simulink model "AJAC_Simulation"  (R2024b)
settings: Solver=FixedStepAuto  StartTime=0.0  StopTime=1  FixedStep=0.000025  RelTol=1e-7  EnableMultiTasking=on
InitFcn:
  | Ld=5.25e-3;
  | Lq=12e-3;
  | R=0.958;
  | f=0.1827;
model workspace (MAT data in the model file):
  f = Simulink.Signal
  f.Dimensions = 1
  f.DimensionsMode = 'auto'
  f.Complexity = 'real'
  f.SampleTime = -1
  f.SamplingMode = 'auto'
  f.InitialValue = '0.1827'
  f.DataType = 'single'
libraries: slpidlib x2, mcbplantlib x1, simulink x1, spsPermanentMagnetSynchronousMachineLib x1, autolibpmsmexterior x1, spspowerguiLib x1
(part 1 of 2)
settings Model: Creator=张豪  LastModifiedBy=ergo
settings SolverCC: AutoInsertRateTranBlk=on
settings DebuggingCC: MultiTaskDSMMsg=none  UnconnectedInputMsg=warning  UnconnectedOutputMsg=warning  UnconnectedLineMsg=warning
settings ModelReferenceCC: EnableRefExpFcnMdlSchedulingChecks=on
settings RTWCC: GPUComputeCapability=3.5  DLArmComputeVersion=19.05

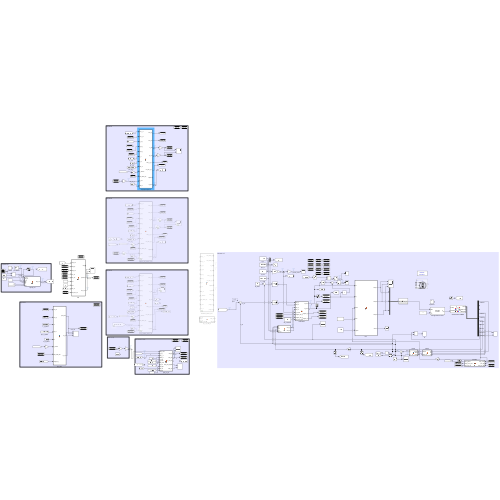
[thumbnail: Simulink's stored preview of the top-level diagram]
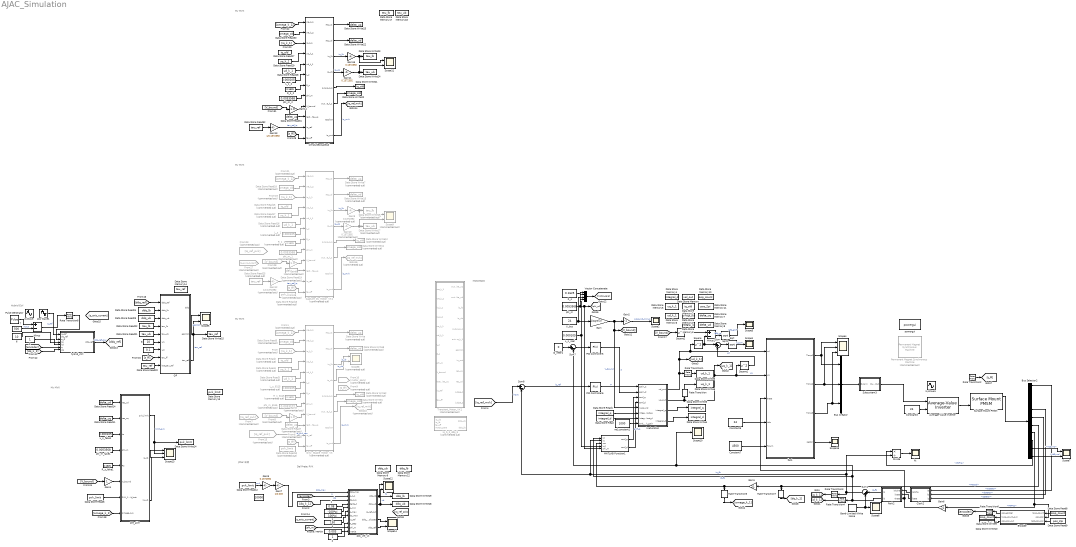
== system AJAC_Simulation ==
  note: jitter 来源
  note: Hybrid Ctrl
  note: My MVK
  note: Del Prete: PVK
  note: Motor8115
  note: My MVK
  note: My MVK
  note: My MVK
  " " : Constant  Value=10000
  "  " : Constant  Value=-100*pi
  " 1" : Constant  Value=0.08
  " 2" : Constant
  " 3" : Constant  Value=100*pi
  " 4" : Constant  Value=150
  " 5" : Constant
  " 6" : Constant  Value=10
  " 7" : Constant  Value=500
  " 8" : Constant  Value=10
  " 9" : Constant  Value=0.1
  Average-Value Inverter : mcbplantlib/Average-Value Inverter
  Band-Limited White Noise : simulink/Sources/Band-Limited White Noise  Cov=[0.0000002]  Ts=0.000025  seed=[23341]
  Bus Creator : BusCreator  Inputs=3
  Bus Selector2 : BusSelector  OutputSignals=IaStator,IqSync,IdSync,IbStator,IcStator,MtrSpd,MtrPos,MtrTrq,VqSync,VdSync
  Capture_Dy_Motor_VK1 : MATLAB Function  Commented=on  TreatAsAtomicUnit=on
  Clark2 : MATLAB Function  TreatAsAtomicUnit=on
  Constant3 : Constant  Value=24
  Constant6 : Constant  Value=24
  Constant7 : Constant  Value=4500  OutDataTypeStr=single
  Data Store Memory : DataStoreMemory  DataStoreName=vel_out  ReadBeforeWriteMsg=warning  WriteAfterWriteMsg=warning  WriteAfterReadMsg=warning  ShowAdditionalParam=off  OutDataTypeStr=double
  Data Store Memory1 : DataStoreMemory  DataStoreName=omega_old  ReadBeforeWriteMsg=warning  WriteAfterWriteMsg=warning  WriteAfterReadMsg=warning  ShowAdditionalParam=off  OutDataTypeStr=double
  Data Store Memory10 : DataStoreMemory  DataStoreName=loop_count  ReadBeforeWriteMsg=warning  WriteAfterWriteMsg=warning  WriteAfterReadMsg=warning  ShowAdditionalParam=off  OutDataTypeStr=double
  Data Store Memory11 : DataStoreMemory  DataStoreName=pos_2pi  ReadBeforeWriteMsg=warning  WriteAfterWriteMsg=warning  WriteAfterReadMsg=warning  ShowAdditionalParam=off  OutDataTypeStr=double
  Data Store Memory12 : DataStoreMemory  DataStoreName=ddq_lb  ReadBeforeWriteMsg=warning  WriteAfterWriteMsg=warning  WriteAfterReadMsg=warning  InitialValue=-1330  ShowAdditionalParam=off  OutDataTypeStr=double
  Data Store Memory13 : DataStoreMemory  DataStoreName=pvk_limit  ReadBeforeWriteMsg=warning  WriteAfterWriteMsg=warning  WriteAfterReadMsg=warning  ShowAdditionalParam=off  OutDataTypeStr=double
  Data Store Memory14 : DataStoreMemory  DataStoreName=tau_ref  ReadBeforeWriteMsg=warning  WriteAfterWriteMsg=warning  WriteAfterReadMsg=warning  ShowAdditionalParam=off  OutDataTypeStr=double
  Data Store Memory17 : DataStoreMemory  DataStoreName=tau_lb  ReadBeforeWriteMsg=warning  WriteAfterWriteMsg=warning  WriteAfterReadMsg=warning  InitialValue=-4  ShowAdditionalParam=off  OutDataTypeStr=double
  Data Store Memory18 : DataStoreMemory  DataStoreName=tau_ub  ReadBeforeWriteMsg=warning  WriteAfterWriteMsg=warning  WriteAfterReadMsg=warning  InitialValue=4  ShowAdditionalParam=off  OutDataTypeStr=double
  Data Store Memory2 : DataStoreMemory  DataStoreName=iq_old  ReadBeforeWriteMsg=warning  WriteAfterWriteMsg=warning  WriteAfterReadMsg=warning  ShowAdditionalParam=off  OutDataTypeStr=double
  Data Store Memory3 : DataStoreMemory  DataStoreName=integral_q  ReadBeforeWriteMsg=warning  WriteAfterWriteMsg=warning  WriteAfterReadMsg=warning  ShowAdditionalParam=off  OutDataTypeStr=double
  Data Store Memory4 : DataStoreMemory  DataStoreName=integral_d  ReadBeforeWriteMsg=warning  WriteAfterWriteMsg=warning  WriteAfterReadMsg=warning  ShowAdditionalParam=off  OutDataTypeStr=double
  Data Store Memory5 : DataStoreMemory  DataStoreName=uq_k_1  ReadBeforeWriteMsg=warning  WriteAfterWriteMsg=warning  WriteAfterReadMsg=warning  ShowAdditionalParam=off  OutDataTypeStr=double
  Data Store Memory6 : DataStoreMemory  DataStoreName=ud_k_1  ReadBeforeWriteMsg=warning  WriteAfterWriteMsg=warning  WriteAfterReadMsg=warning  ShowAdditionalParam=off  OutDataTypeStr=double
  Data Store Memory7 : DataStoreMemory  DataStoreName=delta_uq  ReadBeforeWriteMsg=warning  WriteAfterWriteMsg=warning  WriteAfterReadMsg=warning  ShowAdditionalParam=off  OutDataTypeStr=double
  Data Store Memory8 : DataStoreMemory  DataStoreName=delta_ud  ReadBeforeWriteMsg=warning  WriteAfterWriteMsg=warning  WriteAfterReadMsg=warning  ShowAdditionalParam=off  OutDataTypeStr=double
  Data Store Memory9 : DataStoreMemory  DataStoreName=ddq_ub  ReadBeforeWriteMsg=warning  WriteAfterWriteMsg=warning  WriteAfterReadMsg=warning  InitialValue=1330  ShowAdditionalParam=off  OutDataTypeStr=double
  Data Store Read : DataStoreRead  DataStoreName=integral_d  DataStoreElements=integral_d  IndexOptions=Index vector (dialog)  Indices=1  OutputSizes=1
  Data Store Read1 : DataStoreRead  DataStoreName=integral_q  DataStoreElements=integral_q  IndexOptions=Index vector (dialog)  Indices=1  OutputSizes=1
  Data Store Read10 : DataStoreRead  Commented=on  DataStoreName=pvk_limit  IndexOptions=Index vector (dialog)  Indices=1  OutputSizes=1
  Data Store Read11 : DataStoreRead  DataStoreName=delta_uq  IndexOptions=Index vector (dialog)  Indices=1  OutputSizes=1
  Data Store Read12 : DataStoreRead  DataStoreName=pvk_limit  IndexOptions=Index vector (dialog)  Indices=1  OutputSizes=1
  Data Store Read13 : DataStoreRead  Commented=on  DataStoreName=pvk_limit  IndexOptions=Index vector (dialog)  Indices=1  OutputSizes=1
  Data Store Read14 : DataStoreRead  DataStoreName=delta_ud  IndexOptions=Index vector (dialog)  Indices=1  OutputSizes=1
  Data Store Read15 : DataStoreRead  Commented=on  DataStoreName=iq_old  DataStoreElements=iq_old  IndexOptions=Index vector (dialog)  Indices=1  OutputSizes=1
  Data Store Read16 : DataStoreRead  Commented=on  DataStoreName=ud_k_1  IndexOptions=Index vector (dialog)  Indices=1  OutputSizes=1
  Data Store Read17 : DataStoreRead  Commented=on  DataStoreName=uq_k_1  IndexOptions=Index vector (dialog)  Indices=1  OutputSizes=1
  Data Store Read18 : DataStoreRead  Commented=on  DataStoreName=omega_old  IndexOptions=Index vector (dialog)  Indices=1  OutputSizes=1
  Data Store Read19 : DataStoreRead  Commented=on  DataStoreName=delta_uq  IndexOptions=Index vector (dialog)  Indices=1  OutputSizes=1
  Data Store Read2 : DataStoreRead  Commented=on  DataStoreName=iq_old  DataStoreElements=iq_old  IndexOptions=Index vector (dialog)  Indices=1  OutputSizes=1
  Data Store Read20 : DataStoreRead  DataStoreName=tau_ref  IndexOptions=Index vector (dialog)  Indices=1  OutputSizes=1
  Data Store Read21 : DataStoreRead  DataStoreName=tau_ub  IndexOptions=Index vector (dialog)  Indices=1  OutputSizes=1
  Data Store Read22 : DataStoreRead  DataStoreName=tau_lb  IndexOptions=Index vector (dialog)  Indices=1  OutputSizes=1
  Data Store Read23 : DataStoreRead  DataStoreName=ddq_ub  IndexOptions=Index vector (dialog)  Indices=1  OutputSizes=1
  Data Store Read24 : DataStoreRead  DataStoreName=ddq_lb  IndexOptions=Index vector (dialog)  Indices=1  OutputSizes=1
  Data Store Read25 : DataStoreRead  Commented=on  DataStoreName=tau_ref  IndexOptions=Index vector (dialog)  Indices=1  OutputSizes=1
  Data Store Read27 : DataStoreRead  DataStoreName=iq_old  DataStoreElements=iq_old  IndexOptions=Index vector (dialog)  Indices=1  OutputSizes=1
  Data Store Read28 : DataStoreRead  DataStoreName=ud_k_1  IndexOptions=Index vector (dialog)  Indices=1  OutputSizes=1
  Data Store Read29 : DataStoreRead  DataStoreName=uq_k_1  IndexOptions=Index vector (dialog)  Indices=1  OutputSizes=1
  Data Store Read3 : DataStoreRead  Commented=on  DataStoreName=ud_k_1  IndexOptions=Index vector (dialog)  Indices=1  OutputSizes=1
  Data Store Read30 : DataStoreRead  DataStoreName=omega_old  IndexOptions=Index vector (dialog)  Indices=1  OutputSizes=1
  Data Store Read31 : DataStoreRead  DataStoreName=delta_uq  IndexOptions=Index vector (dialog)  Indices=1  OutputSizes=1
  Data Store Read32 : DataStoreRead  DataStoreName=tau_ref  IndexOptions=Index vector (dialog)  Indices=1  OutputSizes=1
  Data Store Read4 : DataStoreRead  Commented=on  DataStoreName=uq_k_1  IndexOptions=Index vector (dialog)  Indices=1  OutputSizes=1
  Data Store Read5 : DataStoreRead  Commented=on  DataStoreName=omega_old  IndexOptions=Index vector (dialog)  Indices=1  OutputSizes=1
  Data Store Read6 : DataStoreRead  DataStoreName=pvk_limit  IndexOptions=Index vector (dialog)  Indices=1  OutputSizes=1
  Data Store Read7 : DataStoreRead  Commented=on  DataStoreName=delta_uq  IndexOptions=Index vector (dialog)  Indices=1  OutputSizes=1
  Data Store Read8 : DataStoreRead  DataStoreName=loop_count  IndexOptions=Index vector (dialog)  Indices=1  OutputSizes=1
  Data Store Read9 : DataStoreRead  DataStoreName=pos_2pi  IndexOptions=Index vector (dialog)  Indices=1  OutputSizes=1
  Data Store Write : DataStoreWrite  Commented=on  DataStoreName=delta_uq  IndexOptions=Index vector (dialog)  Indices=1  OutputSizes=1
  Data Store Write1 : DataStoreWrite  Commented=on  DataStoreName=omega_old  DataStoreElements=omega_old  IndexOptions=Index vector (dialog)  Indices=1  OutputSizes=1
  Data Store Write10 : DataStoreWrite  DataStoreName=pos_2pi  IndexOptions=Index vector (dialog)  Indices=1  OutputSizes=1
  Data Store Write11 : DataStoreWrite  Commented=on  DataStoreName=omega_old  DataStoreElements=omega_old  IndexOptions=Index vector (dialog)  Indices=1  OutputSizes=1
  Data Store Write12 : DataStoreWrite  Commented=on  DataStoreName=iq_old  DataStoreElements=iq_old  IndexOptions=Index vector (dialog)  Indices=1  OutputSizes=1
  Data Store Write13 : DataStoreWrite  Commented=on  DataStoreName=delta_ud  IndexOptions=Index vector (dialog)  Indices=1  OutputSizes=1
  Data Store Write14 : DataStoreWrite  DataStoreName=pvk_limit  IndexOptions=Index vector (dialog)  Indices=1  OutputSizes=1
  Data Store Write15 : DataStoreWrite  DataStoreName=tau_ref  IndexOptions=Index vector (dialog)  Indices=1  OutputSizes=1
  Data Store Write16 : DataStoreWrite  Commented=on  DataStoreName=tau_lb  IndexOptions=Index vector (dialog)  Indices=1  OutputSizes=1
  Data Store Write17 : DataStoreWrite  Commented=on  DataStoreName=tau_ub  IndexOptions=Index vector (dialog)  Indices=1  OutputSizes=1
  Data Store Write18 : DataStoreWrite  DataStoreName=ddq_ub  IndexOptions=Index vector (dialog)  Indices=1  OutputSizes=1
  Data Store Write19 : DataStoreWrite  DataStoreName=ddq_lb  IndexOptions=Index vector (dialog)  Indices=1  OutputSizes=1
  Data Store Write2 : DataStoreWrite  Commented=on  DataStoreName=iq_old  DataStoreElements=iq_old  IndexOptions=Index vector (dialog)  Indices=1  OutputSizes=1
  Data Store Write20 : DataStoreWrite  DataStoreName=omega_old  DataStoreElements=omega_old  IndexOptions=Index vector (dialog)  Indices=1  OutputSizes=1
  Data Store Write21 : DataStoreWrite  DataStoreName=iq_old  DataStoreElements=iq_old  IndexOptions=Index vector (dialog)  Indices=1  OutputSizes=1
  Data Store Write22 : DataStoreWrite  DataStoreName=delta_ud  IndexOptions=Index vector (dialog)  Indices=1  OutputSizes=1
  Data Store Write23 : DataStoreWrite  DataStoreName=tau_lb  IndexOptions=Index vector (dialog)  Indices=1  OutputSizes=1
  Data Store Write24 : DataStoreWrite  DataStoreName=tau_ub  IndexOptions=Index vector (dialog)  Indices=1  OutputSizes=1
  Data Store Write25 : DataStoreWrite  DataStoreName=delta_uq  IndexOptions=Index vector (dialog)  Indices=1  OutputSizes=1
  Data Store Write3 : DataStoreWrite  DataStoreName=integral_q  DataStoreElements=integral_q  IndexOptions=Index vector (dialog)  Indices=1  OutputSizes=1
  Data Store Write4 : DataStoreWrite  DataStoreName=integral_d  DataStoreElements=integral_d  IndexOptions=Index vector (dialog)  Indices=1  OutputSizes=1
  Data Store Write5 : DataStoreWrite  DataStoreName=ud_k_1  DataStoreElements=ud_k_1  IndexOptions=Index vector (dialog)  Indices=1  OutputSizes=1
  Data Store Write6 : DataStoreWrite  DataStoreName=uq_k_1  DataStoreElements=uq_k_1  IndexOptions=Index vector (dialog)  Indices=1  OutputSizes=1
  Data Store Write7 : DataStoreWrite  Commented=on  DataStoreName=delta_uq  IndexOptions=Index vector (dialog)  Indices=1  OutputSizes=1
  Data Store Write8 : DataStoreWrite  Commented=on  DataStoreName=delta_ud  IndexOptions=Index vector (dialog)  Indices=1  OutputSizes=1
  Data Store Write9 : DataStoreWrite  DataStoreName=loop_count  IndexOptions=Index vector (dialog)  Indices=1  OutputSizes=1
  Divide : Product  Inputs=*/
  Encoder : MATLAB Function  TreatAsAtomicUnit=on
  From : From  Commented=on  GotoTag=iq_k_1
  From1 : From  Commented=on  GotoTag=omega_k_1
  From10 : From  Commented=on  GotoTag=motor_para
  From13 : From  Commented=on  GotoTag=iq_ref_pvk
  From19 : From  Commented=on  GotoTag=iq_k_1
  From21 : From  Commented=on  GotoTag=omega_k_1
  From23 : From  Commented=on  GotoTag=iq_ref_pvk
  From26 : From  Commented=on  GotoTag=t_ff
  From27 : From  Commented=on  GotoTag=q_axis_current
  From28 : From  Commented=on  GotoTag=V_bound
  From6 : From  Commented=on  GotoTag=t_ff
  From7 : From  Commented=on  GotoTag=iq_ref_pvk
  From8 : From  Commented=on  GotoTag=V_bound
  From9 : From  Commented=on  GotoTag=t_ff
  Gain : Gain  Gain=1/sqrt(3)
  Gain1 : Gain  Gain=21
  Gain10 : Gain  Commented=on  Gain=0.1372392
  Gain11 : Gain  Gain=0.1372392
  Gain12 : Gain  Commented=on  Gain=1/0.1372392
  Gain13 : Gain  Gain=1/0.1372392
  Gain14 : Gain  Gain=1.0
  Gain15 : Gain  Gain=0.1372392
  Gain2 : Gain  Gain=-1
  Gain3 : Gain  Commented=on  Gain=1.0
  Gain4 : Gain
  Gain5 : Gain  Gain=0.1372392
  Gain6 : Gain  Gain=21
  Gain7 : Gain  Gain=1/0.003
  Gain8 : Gain  Commented=on  Gain=1.0
  Gain9 : Gain  Commented=on  Gain=0.1372392
  Goto10 : Goto  Commented=on  GotoTag=iq_ref_mvk
  Goto16 : Goto  Commented=on  GotoTag=iq_ref_mvk
  I saturation : MATLAB Function  TreatAsAtomicUnit=on
  L_s_1 : Constant  Commented=on  Value=0.000105
  L_s_2 : Constant  Value=0.000105
  L_s_8115 : Constant  Commented=on  Value=0.000105
  L_s_fake1 : Constant  Value=0.000105
  L_s_real : Constant  Value=0.000105
  MATLAB Function1 : MATLAB Function  TreatAsAtomicUnit=on
  Minus : Sum  Inputs=+-
  Minus1 : Sum  Inputs=+-
  Only_Stable_Motor_VK : MATLAB Function  Commented=on  TreatAsAtomicUnit=on
  PID Controller5 : slpidlib/PID Controller  Controller=P  Form=Ideal  TimeDomain=Discrete-time  UseExternalTs=off  SampleTime=-1  IntegratorMethod=Forward Euler  FilterMethod=Forward Euler  ControllerParametersSource=internal  P=1.2  I=1614.8  UseKiTs=off  D=0  UseExternalDerivativeSource=off  N=100  UseFilter=on  TunerSelectOption=Transfer Function Based (PID Tuner App)  InitialConditionSource=internal  InitialConditionForIntegrator=0  InitialConditionForFilter=0  DifferentiatorICPrevScaledInput=0  ExternalReset=none  TrackingMode=off  Kt=1  LimitOutput=on  SatLimitsSource=internal  UpperSaturationLimit=36  LowerSaturationLimit=-36  LinearizeAsGain=on  AntiWindupMode=none  Kb=1  LimitIntegrator=off  UpperIntegratorSaturationLimit=inf  LowerIntegratorSaturationLimit=-inf  POutMin=[]  POutMax=[]  IOutMin=[]  IOutMax=[]  DOutMin=[]  DOutMax=[]  NOutMin=[]  NOutMax=[]  SumOutMin=[]  SumOutMax=[]  SaturationOutMin=[]  SaturationOutMax=[]  PParamMin=[]  PParamMax=[]  IParamMin=[]  IParamMax=[]  DParamMin=[]  DParamMax=[]  NParamMin=[]  NParamMax=[]  KbParamMin=[]  KbParamMax=[]  KtParamMin=[]  KtParamMax=[]  KbOutMin=[]  KbOutMax=[]  KtOutMin=[]  KtOutMax=[]  IntegratorOutMin=[]  IntegratorOutMax=[]  FilterOutMin=[]  FilterOutMax=[]  SumI1OutMin=[]  SumI1OutMax=[]  SumI2OutMin=[]  SumI2OutMax=[]  SumI3OutMin=[]  SumI3OutMax=[]  SumI4OutMin=[]  SumI4OutMax=[]  SumDOutMin=[]  SumDOutMax=[]  DifferentiatorOutMin=[]  DifferentiatorOutMax=[]  FilterDiffOutCoefMin=[]  FilterDiffOutCoefMax=[]  ReciprocalOutMin=[]  ReciprocalOutMax=[]  SumDenOutMin=[]  SumDenOutMax=[]  SumNumOutMin=[]  SumNumOutMax=[]  DivideOutMin=[]  DivideOutMax=[]  UdiffTsProdOutMin=[]  UdiffTsProdOutMax=[]  NTsProdOutMin=[]  NTsProdOutMax=[]  UintegralTsProdOutMin=[]  UintegralTsProdOutMax=[]  UngainTsProdOutMin=[]  UngainTsProdOutMax=[]  ClampingZeroOutDataTypeStr=Inherit: Inherit via back propagation  ClampingZeroOutMin=[]  ClampingZeroOutMax=[]  FilterDenConstantOutDataTypeStr=Inherit: Inherit via back propagation  FilterDenConstantOutMin=[]  FilterDenConstantOutMax=[]  PCopyOutDataTypeStr=Inherit: Inherit via back propagation  PCopyOutMin=[]  PCopyOutMax=[]  NCopyOutDataTypeStr=Inherit: Inherit via back propagation  NCopyOutMin=[]  NCopyOutMax=[]  IntegratorContinuousStateAttributes=''  IntegratorStateMustResolveToSignalObject=off  IntegratorRTWStateStorageClass=Auto  FilterContinuousStateAttributes=''  FilterStateMustResolveToSignalObject=off  FilterRTWStateStorageClass=Auto  ParallelPVariant=InternalParameters  IdealPVariant=Disabled  IVariant=Disabled  DVariant=Disabled  IntegratorVariant=Disabled  SatVariant=Enabled  AWVariant=Disabled  PCopyVariant=Disabled  TRVariant=Disabled  FdbkBlocksVariant=Forward  IdealPFdbkVariant=Disabled  SatFdbkVariant=Disabled  DerivativeFilterVariant=Disabled  NVariant=Disabled  NCopyVariant=Disabled_SignalSpec  FilterICVariant=Disabled  IntegratorICVariant=Disabled  ExternalResetVariant=Disabled  TRSumVariant=Passthrough  SumFdbkVariant=Disabled  SumVariant=Passthrough_P  TsampFilterVariant=InternalTs  TsampNgainVariant=Passthrough  TsampIntegralVariant=Disabled_SignalSpec  ExternalSaturationOutDataTypeStr=Inherit: Same as second input  DerivativeSourceVariant=Disabled  PreIntVariant=InternalPreInt
  PID Controller6 : slpidlib/PID Controller  Controller=P  Form=Ideal  TimeDomain=Discrete-time  UseExternalTs=off  SampleTime=-1  IntegratorMethod=Forward Euler  FilterMethod=Forward Euler  ControllerParametersSource=internal  P=1.2  I=1614.8  UseKiTs=off  D=0  UseExternalDerivativeSource=off  N=100  UseFilter=on  TunerSelectOption=Transfer Function Based (PID Tuner App)  InitialConditionSource=internal  InitialConditionForIntegrator=0  InitialConditionForFilter=0  DifferentiatorICPrevScaledInput=0  ExternalReset=none  TrackingMode=off  Kt=1  LimitOutput=on  SatLimitsSource=internal  UpperSaturationLimit=36  LowerSaturationLimit=-36  LinearizeAsGain=on  AntiWindupMode=none  Kb=1  LimitIntegrator=off  UpperIntegratorSaturationLimit=inf  LowerIntegratorSaturationLimit=-inf  POutMin=[]  POutMax=[]  IOutMin=[]  IOutMax=[]  DOutMin=[]  DOutMax=[]  NOutMin=[]  NOutMax=[]  SumOutMin=[]  SumOutMax=[]  SaturationOutMin=[]  SaturationOutMax=[]  PParamMin=[]  PParamMax=[]  IParamMin=[]  IParamMax=[]  DParamMin=[]  DParamMax=[]  NParamMin=[]  NParamMax=[]  KbParamMin=[]  KbParamMax=[]  KtParamMin=[]  KtParamMax=[]  KbOutMin=[]  KbOutMax=[]  KtOutMin=[]  KtOutMax=[]  IntegratorOutMin=[]  IntegratorOutMax=[]  FilterOutMin=[]  FilterOutMax=[]  SumI1OutMin=[]  SumI1OutMax=[]  SumI2OutMin=[]  SumI2OutMax=[]  SumI3OutMin=[]  SumI3OutMax=[]  SumI4OutMin=[]  SumI4OutMax=[]  SumDOutMin=[]  SumDOutMax=[]  DifferentiatorOutMin=[]  DifferentiatorOutMax=[]  FilterDiffOutCoefMin=[]  FilterDiffOutCoefMax=[]  ReciprocalOutMin=[]  ReciprocalOutMax=[]  SumDenOutMin=[]  SumDenOutMax=[]  SumNumOutMin=[]  SumNumOutMax=[]  DivideOutMin=[]  DivideOutMax=[]  UdiffTsProdOutMin=[]  UdiffTsProdOutMax=[]  NTsProdOutMin=[]  NTsProdOutMax=[]  UintegralTsProdOutMin=[]  UintegralTsProdOutMax=[]  UngainTsProdOutMin=[]  UngainTsProdOutMax=[]  ClampingZeroOutDataTypeStr=Inherit: Inherit via back propagation  ClampingZeroOutMin=[]  ClampingZeroOutMax=[]  FilterDenConstantOutDataTypeStr=Inherit: Inherit via back propagation  FilterDenConstantOutMin=[]  FilterDenConstantOutMax=[]  PCopyOutDataTypeStr=Inherit: Inherit via back propagation  PCopyOutMin=[]  PCopyOutMax=[]  NCopyOutDataTypeStr=Inherit: Inherit via back propagation  NCopyOutMin=[]  NCopyOutMax=[]  IntegratorContinuousStateAttributes=''  IntegratorStateMustResolveToSignalObject=off  IntegratorRTWStateStorageClass=Auto  FilterContinuousStateAttributes=''  FilterStateMustResolveToSignalObject=off  FilterRTWStateStorageClass=Auto  ParallelPVariant=InternalParameters  IdealPVariant=Disabled  IVariant=Disabled  DVariant=Disabled  IntegratorVariant=Disabled  SatVariant=Enabled  AWVariant=Disabled  PCopyVariant=Disabled  TRVariant=Disabled  FdbkBlocksVariant=Forward  IdealPFdbkVariant=Disabled  SatFdbkVariant=Disabled  DerivativeFilterVariant=Disabled  NVariant=Disabled  NCopyVariant=Disabled_SignalSpec  FilterICVariant=Disabled  IntegratorICVariant=Disabled  ExternalResetVariant=Disabled  TRSumVariant=Passthrough  SumFdbkVariant=Disabled  SumVariant=Passthrough_P  TsampFilterVariant=InternalTs  TsampNgainVariant=Passthrough  TsampIntegralVariant=Disabled_SignalSpec  ExternalSaturationOutDataTypeStr=Inherit: Same as second input  DerivativeSourceVariant=Disabled  PreIntVariant=InternalPreInt
  Park2 : MATLAB Function  TreatAsAtomicUnit=on
  Permanent Magnet Synchronous Machine : spsPermanentMagnetSynchronousMachineLib/Permanent Magnet Synchronous Machine  Commented=on  NbPhases=3  FluxDistribution=Sinusoidal  RotorType=Round  MechanicalLoad=Torque Tm  PresetModel=No  ShowDetailedParameters=on  MeasurementBus=off  Resistance=0.073  Inductance=8.5e-3  dqInductances=[8.5e-3,8.5e-3]  La=8.65e-05  MachineConstant=Flux linkage established by magnets (V.s)  Flux=0.00941775  VoltageCst=35.872  TorqueCst=0.29666  Flat=120  Mechanical=[0.00120108 3.03448e-06 21]  PolePairs=4  InitialConditions=[0,0, 0,0]  InitialConditions5ph=[0 0 0 0 0 0]  RefAngle=90 degrees behind phase A axis (modified Park)  IterativeDiscreteModel=Trapezoidal non iterative  TsBlock=-1  TsPowergui=0
  Pulse Generator : DiscretePulseGenerator  PulseType=Time based  Amplitude=1000  Period=0.5  PulseWidth=50
  QP : MATLAB Function  TreatAsAtomicUnit=on
  R_s : Constant  Value=0.1625
  R_s_1 : Constant  Commented=on  Value=0.1625
  R_s_2 : Constant  Value=0.1625
  R_s_8115 : Constant  Commented=on  Value=0.1625
  R_s_fake1 : Constant  Value=0.1625
  Rate Transition{,1..8} (9 alike) : RateTransition  OutPortSampleTime=0.001
  Scope{1..3,6,10,16} (6 alike) : Scope
  Scope{5,7,11..12,14} (5 alike) : Scope  NumInputPorts=2
  Scope13 : Scope  NumInputPorts=3
  Scope4 : Scope  NumInputPorts=3
  Scope8 : Scope  Commented=on  NumInputPorts=2
  Scope9 : Scope  Commented=on  NumInputPorts=2
  Sqrt : Sqrt
  Sqrt1 : Sqrt
  Square : Math  Operator=square
  Square1 : Math  Operator=square
  Square2 : Math  Operator=square
  Subsystem3 : Subsystem
  Sum : Sum  Inputs=|++
  Sum1 : Sum  Inputs=|++
  Sum7 : Sum  Inputs=|+-
  Sum8 : Sum  Inputs=|+-
  Surface Mount PMSM : autolibpmsmexterior/Surface Mount PMSM  port_config=Torque  sim_type=Continuous  Ts=0.0000025  FilePath=motor_model  P=21  Rs=0.1625  Ldq_=0.000105  KConstText=Permanent flux linkage constant (lambda_pm):  lambda_pm=0.0043568  Ke=22.755  Kt=0.22317  mechanical=[0.0003,0.001, 0.1]  idq0=[0 0]  theta_init=0  omega_init=0  KConst=0.0043568  lambda_pm_calc=0.0043568  RefBlkName='autolibpmsmexterior/Surface Mount PMSM'  aMode=5  Ldq="[0.0017      0.0017]"
  Transient_Motor_VK1 : MATLAB Function  Commented=on  TreatAsAtomicUnit=on
  V_bus : Constant  Value=24  OutDataTypeStr=double
  Vector Concatenate : Concatenate  NumInputs=4
  foc1 : MATLAB Function  TreatAsAtomicUnit=on
  hybrid_ctrl : MATLAB Function  TreatAsAtomicUnit=on
  id_refer1 : Constant  Value=0
  inertia : Constant  Value=0.003
  iq Wave : Sin  Amplitude=30  Frequency=10  SampleTime=0
  iq Wave1 : Sin  Amplitude=2  Frequency=10  SampleTime=0
  iq_b_2_ddq_b : MATLAB Function  Commented=on  TreatAsAtomicUnit=on
  kt : Scope
  phi_m : Constant  Value=0.0053568
  phi_m_1 : Constant  Commented=on  Value=0.0053568
  phi_m_2 : Constant  Value=0.0053568
  phi_m_8115 : Constant  Commented=on  Value=0.0053568
  phi_m_fake1 : Constant  Value=0.0053568
  pos Wave1 : Sin  Amplitude=20  Frequency=40  SampleTime=0
  pos_vel_vk : MATLAB Function  TreatAsAtomicUnit=on
  powergui : spspowerguiLib/powergui  Priority=1  SimulationMode=Discrete  SampleTime=0.000025  frequency=60  Iterations=50  frequencyindice=0  Pbase=100e6  ErrMax=1e-4  UnitsV=kV  UnitsW=MW  buscounter=0  FunctionMessages=off  echomessages=off  EnableUseOfTLC=off  CurrentSourceSwitches=off  DisableSnubberDevices=off  DisableRonSwitches=off  DisableVfSwitches=off  DisplayEquations=off  AutomaticDiscreteSolvers=off  SolverType=Tustin/Backward Euler (TBE)  Interpol=off  ExternalGateDelay=off  methode=off  Ts=100  x0status=blocks  SPID=on  SwTol=0  HookPort=off  NonlinearTolerance=1e-4  nMaxIteration=100  ContinueOnMaxIteration=off  RestoreLinks=warning  ResistiveCurrentMeasurement=off  Frange=[0:2:500]  Ylog=off  Xlog=on  ShowGrid=off  save=off  variable=ZData  structure=0  ZoomFFT=off  StartTime=0.0  cycles=1  DisplayStyle=1  fundamental=60  FreqAxis=off  MaxFrequency=1000  frequencyindicesteady=1  RmsSteady=1  display=off
  pre_alim : MATLAB Function  TreatAsAtomicUnit=on
  ref_constant1 : Constant  Value=1000
  simplydecoupleud : MATLAB Function  TreatAsAtomicUnit=on
  wires:
  Only_Stable_Motor_VK/5(out_iq_k_1) -> Data Store Write2/1
  Only_Stable_Motor_VK/6(out_we_k_1) -> Data Store Write1/1
  Only_Stable_Motor_VK/1(res_uq) -> Data Store Write/1
  Only_Stable_Motor_VK/2(res_ud) -> Data Store Write8/1
  Data Store Read7/1 -> Only_Stable_Motor_VK/10(last_delta_uq)
  L_s_8115/1 -> Only_Stable_Motor_VK/6(L_s)
  phi_m_8115/1 -> Only_Stable_Motor_VK/8(phi_m)
  R_s_8115/1 -> Only_Stable_Motor_VK/7(R_s)
  " 4"/1 -> pos_vel_vk/7(dq_max)
  " 3"/1 -> pos_vel_vk/6(q_max)
  "  "/1 -> pos_vel_vk/5(q_min)
  " 1"/1 -> pos_vel_vk/4(delta_t)
  pos_vel_vk/1(ddq_lb) -> Data Store Write19/1, Scope12/1  "lb"
  pos_vel_vk/2(ddq_ub) -> Data Store Write18/1, Scope12/2  "ub"
  inertia/1 -> pos_vel_vk/11(inertia)
  pos_vel_vk/5(ddq_ref) -> Scope14/2
  pos_vel_vk/4(ddq_ref_clipped) -> Scope14/1
  From/1 -> Only_Stable_Motor_VK/3(iq_k_1)
  From1/1 -> Only_Stable_Motor_VK/1(we_k_1)
  Data Store Read9/1 -> Encoder/3(last_pos_2pi)
  Bus Selector2/8 -> Divide/1  "<MtrTrq>"
  phi_m/1 -> Vector Concatenate/2, MATLAB Function1/5(phi_m), [phi_m]
  L_s_real/1 -> Vector Concatenate/4, MATLAB Function1/4(L_s)
  id_refer1/1 -> Sum7/1
  Band-Limited White Noise/1 -> Scope6/1, Sum1/2
  Bus Selector2/5 -> Clark2/3(ic)  "<IcStator>"
  Bus Selector2/1 -> Clark2/1(ia)  "<IaStator>"
  ref_constant1/1 -> I saturation/8(anti_back_gain)
  I saturation/4(integral_d) -> Data Store Write4/1
  foc1/3(Tcmp3) -> Bus Creator/3, Scope4/3
  Surface Mount PMSM/1 -> Bus Selector2/1
  Park2/2(id) -> Scope10/1, Sum7/2, MATLAB Function1/1(id), Rate Transition4/1  "id_fb"
  Constant6/1 -> foc1/4(Udc)
  Sum7/1 -> PID Controller5/1
  Encoder/3(pos_2pi_out) -> Data Store Write10/1
  I saturation/1(ud_out) -> Rate Transition1/1, [ud_k_1], Square/1, foc1/1(ud)  "ud"
  PID Controller5/1 -> I saturation/2(gain_d)  "p"
  Sum1/1 -> Sum8/2, MATLAB Function1/2(iq), Divide/2, Rate Transition3/1  "iq_fb"
  V_bus/1 -> Gain/1, Vector Concatenate/3
  Bus Selector2/4 -> Clark2/2(ib)  "<IbStator>"
  Clark2/1(ialpha) -> Park2/1(ialpha)
  Clark2/2(ibeta) -> Park2/2(ibeta)
  Divide/1 -> kt/1
  I saturation/2(uq_out) -> Square1/1, foc1/2(uq), [uq_k_1], Rate Transition/1  "uq"
  Bus Selector2/7 -> Encoder/2(pos_2pi), Gain6/1  "<MtrPos>"
  MATLAB Function1/2(emf_d) -> I saturation/4(emf_d)
  Data Store Read8/1 -> Encoder/1(loop_count)
  Subsystem3/1(DutyOut) -> Average-Value Inverter/1
  foc1/2(Tcmp2) -> Bus Creator/2, Scope4/2
  Bus Selector2/9 -> Scope7/1  "<VqSync>"
  Gain6/1 -> foc1/3(theta), Park2/3(theta)
  I saturation/3(integral_q) -> Data Store Write3/1
  Data Store Read/1 -> I saturation/7(integral_last_d)
  PID Controller6/1 -> I saturation/1(gain_q)  "P"
  Park2/1(iq) -> Sum1/1  "iq_fb"
  Sum8/1 -> PID Controller6/1  "iq_ref"
  Constant7/1 -> foc1/5(Tpwm)
  MATLAB Function1/1(emf_q) -> I saturation/3(emf_q)  "emf_q"
  Bus Selector2/10 -> Scope7/2  "<VdSync>"
  foc1/4(sector) -> Scope16/1
  Average-Value Inverter/1 -> Surface Mount PMSM/2
  Data Store Read1/1 -> I saturation/6(integral_last_q)
  Constant3/1 -> Average-Value Inverter/2
  Encoder/2(loop_count_out) -> Data Store Write9/1
  Bus Creator/1 -> Subsystem3/1(DutyIn)
  Gain1/1 -> MATLAB Function1/3(we), Rate Transition5/1
  foc1/1(Tcmp1) -> Bus Creator/1, Scope4/1
  Bus Selector2/6 -> Gain1/1, Rate Transition7/1  "<MtrSpd>"
  [dq_k_1] -> pos_vel_vk/3(dq_k_1)  "dq"
  [encoder] -> pos_vel_vk/2(q_k_1)  "q"
  Only_Stable_Motor_VK/8(iq_out) -> Goto10/1  "iq_mvk"
  [phi_m] -> pos_vel_vk/10(phi_m)
  From6/1 -> Only_Stable_Motor_VK/12(tau_ff)
  Gain/1 -> Gain2/1, [V_bound], I saturation/5(V_bound)  "V_bound"
  Only_Stable_Motor_VK/3(iq_lb) -> Scope8/2  "iq_lb"
  Only_Stable_Motor_VK/4(iq_ub) -> Scope8/1  "iq_ub"
  R_s/1 -> Vector Concatenate/1
  Vector Concatenate/1 -> [motor_para]
  [encoder] -> hybrid_ctrl/6(q)
  [dq_k_1] -> hybrid_ctrl/7(dq)
  From13/1 -> Only_Stable_Motor_VK/11(iq_ref)  "iq_pvk_raw"
  " 2"/1 -> pos_vel_vk/9(N_step)
  Square/1 -> Minus1/2, Sum/1
  Square1/1 -> Sum/2
  Sum/1 -> Sqrt/1
  Sqrt/1 -> Scope1/1  "V_sum"
  Pulse Generator/1 -> Minus/1  "input"
  " 7"/1 -> Minus/2
  Gain2/1 -> Scope2/1  "V_bound_minus"
  [V_bound] -> Square2/1
  Square2/1 -> Minus1/1
  Minus1/1 -> Sqrt1/1  "left_uq"
  Sqrt1/1 -> Scope3/1  "left_emf"
  Data Store Read3/1 -> Only_Stable_Motor_VK/5(ud_k_1)
  Rate Transition/1 -> Data Store Write6/1
  Rate Transition1/1 -> Data Store Write5/1
  Rate Transition2/1 -> [t_ff]
  Rate Transition3/1 -> [iq_k_1]
  Rate Transition4/1 -> [id_k_1]
  Rate Transition5/1 -> [omega_k_1]
  Data Store Read4/1 -> Only_Stable_Motor_VK/4(uq_k_1)
  Encoder/1(pos_global) -> Rate Transition6/1
  Rate Transition6/1 -> [encoder]
  Rate Transition7/1 -> [dq_k_1]
  From8/1 -> Gain3/1
  Gain3/1 -> Only_Stable_Motor_VK/9(V_bound)
  Data Store Read5/1 -> Only_Stable_Motor_VK/2(we_k_2)
  [V_bound] -> Gain4/1
  Data Store Read14/1 -> pre_alim/1(res_ud)
  Data Store Read11/1 -> pre_alim/2(res_uq)
  L_s_fake1/1 -> pre_alim/3(Ls)
  R_s_fake1/1 -> pre_alim/5(Rs)
  phi_m_fake1/1 -> pre_alim/4(phi_m)
  Gain4/1 -> pre_alim/6(V_bound)
  Data Store Read6/1 -> pre_alim/7(PVK_limit_last)
  pre_alim/1(pvk_limit) -> Scope13/2, Data Store Write14/1  "limit_pvk"
  [omega_k_1] -> pre_alim/8(omega_k_1)
  pre_alim/2(iq_lb) -> Scope13/1
  pre_alim/3(iq_ub) -> Scope13/3
  Data Store Read12/1 -> Gain5/1  "pvk"
  Gain5/1 -> Gain7/1
  Gain7/1 -> pos_vel_vk/1(ddq_max)  "ddq_max"
  Minus/1 -> Rate Transition8/1
  Capture_Dy_Motor_VK1/2(res_ud) -> Data Store Write13/1
  Capture_Dy_Motor_VK1/6(out_we_k_1) -> Data Store Write11/1
  From28/1 -> Gain8/1
  Capture_Dy_Motor_VK1/8(iq_out) -> Goto16/1  "iq_mvk"
  Capture_Dy_Motor_VK1/3(iq_lb) -> Gain9/1  "iq_lb"
  L_s_1/1 -> Capture_Dy_Motor_VK1/6(L_s)
  Data Store Read19/1 -> Capture_Dy_Motor_VK1/10(last_delta_uq)
  Gain8/1 -> Capture_Dy_Motor_VK1/9(V_bound)
  Capture_Dy_Motor_VK1/5(out_iq_k_1) -> Data Store Write12/1
  Data Store Read18/1 -> Capture_Dy_Motor_VK1/2(we_k_2)
  From21/1 -> Capture_Dy_Motor_VK1/1(we_k_1)
  Capture_Dy_Motor_VK1/4(iq_ub) -> Gain10/1  "iq_ub"
  R_s_1/1 -> Capture_Dy_Motor_VK1/7(R_s)
  Data Store Read17/1 -> Capture_Dy_Motor_VK1/4(uq_k_1)
  Capture_Dy_Motor_VK1/1(res_uq) -> Data Store Write7/1
  From26/1 -> Capture_Dy_Motor_VK1/12(tau_ff)
  Data Store Read16/1 -> Capture_Dy_Motor_VK1/5(ud_k_1)
  From19/1 -> Capture_Dy_Motor_VK1/3(iq_k_1)
  phi_m_1/1 -> Capture_Dy_Motor_VK1/8(phi_m)
  Data Store Read20/1 -> QP/9(last_tau_ref)
  QP/3(tau_ref) -> Scope5/2, Data Store Write15/1  "tau_ref"
  " 8"/1 -> QP/6(w1)
  " 9"/1 -> QP/7(w2)
  [t_ff] -> QP/8(tau_ff)
  Gain10/1 -> Scope9/2, Data Store Write17/1
  Gain9/1 -> Scope9/1, Data Store Write16/1
  Data Store Read21/1 -> QP/5(tau_ub)
  Data Store Read22/1 -> QP/4(tau_lb)
  Data Store Read24/1 -> QP/2(ddq_lb)
  Data Store Read23/1 -> QP/3(ddq_ub)
  Data Store Read25/1 -> Gain12/1
  Gain12/1 -> Capture_Dy_Motor_VK1/11(iq_ref)  "tau_ref_iq"
  QP/2(epsilon) -> Scope5/1  "epsilon"
  pos Wave1/1 -> hybrid_ctrl/1(q_ref)  "q_ref"
  hybrid_ctrl/1(ddq_ref) -> [ddq_ref]  "ddq_ref_raw"
  [ddq_ref] -> QP/1(ddq_ref)
  " 6"/1 -> hybrid_ctrl/4(kp)
  " 5"/1 -> hybrid_ctrl/5(kd)
  Rate Transition8/1 -> hybrid_ctrl/3(a_ff)
  [iq_ref_mvk] -> Sum8/1  "input"
  phi_m_2/1 -> simplydecoupleud/8(phi_m)
  Data Store Read32/1 -> Gain13/1
  Gain14/1 -> simplydecoupleud/9(V_bound)
  simplydecoupleud/1(res_uq) -> Data Store Write25/1
  Gain15/1 -> Scope11/1, Data Store Write23/1
  simplydecoupleud/4(iq_ub) -> Gain11/1  "iq_ub"
  R_s_2/1 -> simplydecoupleud/7(R_s)
  Data Store Read29/1 -> simplydecoupleud/4(uq_k_1)
  simplydecoupleud/8(iq_out) -> [iq_ref_mvk]  "iq_mvk"
  [omega_k_1] -> simplydecoupleud/1(we_k_1)
  L_s_2/1 -> simplydecoupleud/6(L_s)
  simplydecoupleud/2(res_ud) -> Data Store Write22/1
  simplydecoupleud/3(iq_lb) -> Gain15/1  "iq_lb"
  simplydecoupleud/6(out_we_k_1) -> Data Store Write20/1
  [iq_k_1] -> simplydecoupleud/3(iq_k_1)
  Data Store Read31/1 -> simplydecoupleud/10(last_delta_uq)
  Gain13/1 -> simplydecoupleud/11(iq_ref)  "tau_ref_iq"
  Data Store Read28/1 -> simplydecoupleud/5(ud_k_1)
  simplydecoupleud/5(out_iq_k_1) -> Data Store Write21/1
  Data Store Read30/1 -> simplydecoupleud/2(we_k_2)
  Gain11/1 -> Scope11/2, Data Store Write24/1
  [V_bound] -> Gain14/1
  [t_ff] -> simplydecoupleud/12(tau_ff)

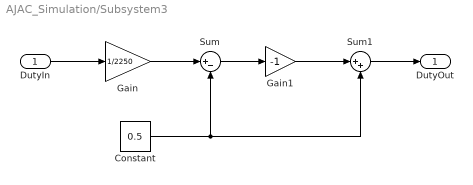
== system AJAC_Simulation/Subsystem3 ==
  DutyIn : Inport
  Constant : Constant  Value=0.5  SampleTime=-1
  Gain : Gain  Gain=1/2250  ParamDataTypeStr=single
  Gain1 : Gain  Gain=-1
  Sum : Sum  Inputs=|+-
  Sum1 : Sum  Inputs=|++
  DutyOut : Outport
  wires:
  Sum/1 -> Gain1/1
  Constant/1 -> Sum1/2, Sum/2
  DutyIn/1 -> Gain/1
  Gain1/1 -> Sum1/1
  Sum1/1 -> DutyOut/1
  Gain/1 -> Sum/1

== matlab function AJAC_Simulation/iq_b_2_ddq_b ==
  settings: updateMethod=DISCRETE  sampleTime=0.001
  data: ddq_ub output; ddq_lb output; iq_ub input; iq_lb input; f data_store_memory; tau_ff input; motor_para input
function [ddq_ub, ddq_lb] = fcn(iq_ub, iq_lb, tau_ff, motor_para)
% 需要注意lb用来减速，ub用来加速。motor_para: r_s, phi_m, V, L_s
inertial = 0.0003;
ddq_ub = (1.5 * motor_para(2)*21 * iq_ub - tau_ff) / inertial;
ddq_lb = (1.5 * motor_para(2)*21 * iq_lb - tau_ff) / inertial;

== matlab function AJAC_Simulation/I saturation ==
  settings: updateMethod=DISCRETE  sampleTime=0.000025
  data: ud_out output; uq_out output; gain_q input; gain_d input; emf_q input; emf_d input; V_bound input; integral_last_q input; integral_last_d input; integral_q output; integral_d output; anti_back_gain input
function [ud_out,uq_out, integral_q, integral_d]  = fcn(gain_q, gain_d, emf_q, emf_d, V_bound, integral_last_q, integral_last_d, anti_back_gain)

integral_raw_d = integral_last_d + gain_d * 1547.6190476190 * 0.000025;
u_d_raw = gain_d + emf_d + integral_raw_d;

integral_raw_q = integral_last_q + gain_q * 1547.6190476190* 0.000025;
u_q_raw = gain_q + emf_q + integral_raw_q;

voltage_line = sqrt(u_q_raw* u_q_raw + u_d_raw * u_d_raw);

if(voltage_line > V_bound)
    if(abs(u_d_raw) > V_bound)
        ud_out = sign(u_d_raw) * V_bound;
    else
        ud_out = u_d_raw;
    end
    uq_out = sign(u_q_raw) *sqrt(V_bound* V_bound - ud_out* ud_out);
else
    ud_out = u_d_raw;
    uq_out = u_q_raw;
end

integral_q = integral_raw_q + ( anti_back_gain*(uq_out - u_q_raw))*0.000025;
integral_d = integral_raw_d + (anti_back_gain*(ud_out - u_d_raw))*0.000025;
% integral_q = integral_raw_q;
% integral_d = integral_raw_d;



% 抗饱和，因为积分会一直积累误差。
% 问题在于很大速度减速不wok
% sat_q = pi_p_q + emf_q;
% sat_d = pi_p_d + emf_d;
% 
% sat_lb_q = min([0, -V_bound - sat_q]);
% sat_ub_q = max([0, V_bound - sat_q]);
% 
% sat_lb_d = min([0, -V_bound- sat_d]);
% sat_ub_d = max([0, V_bound - sat_d]);

% if(we*pi_p_q > 0) && (pi_i_q > V_bound)
%     is_sat = 1;
%     signal = 0;
% end
% 
% if(we * pi_p_q < 0)
%     is_sat = 0;
%     signal = 0;
% end

== matlab function AJAC_Simulation/hybrid_ctrl ==
  settings: updateMethod=DISCRETE  sampleTime=0.001
  data: ddq_ref output; q_ref input; dq_ref input; f data_store_memory; a_ff input; kp input; kd input; q input; dq input
function ddq_ref  = fcn(q_ref, dq_ref, a_ff, kp, kd, q, dq)
% 需要注意lb用来减速，ub用来加速。motor_para: r_s, phi_m, V, L_s
ddq_ref = kp * (q_ref - q) + kd* (dq_ref - dq) + a_ff;

== matlab function AJAC_Simulation/MATLAB Function1 ==
  settings: updateMethod=DISCRETE  sampleTime=0.000025
  data: id input; iq input; we input; f data_store_memory; emf_q output; emf_d output; L_s input; phi_m input
function [emf_q,emf_d] = fcn(id,iq, we,L_s,phi_m)
emf_q = we *(phi_m+L_s*id);
emf_d = -we*iq*L_s;

== matlab function AJAC_Simulation/Transient_Motor_VK1 ==
  settings: updateMethod=DISCRETE  sampleTime=0.001
  data: out_delta_uq output; out_delta_ud output; we_k_1 input; we_k_2 input; iq_k_1 input; iq_k_2 input; uq_k_1 input; ud_k_1 input; L_s input; R_s input; f data_store_memory; iq_lb output; iq_ub output; phi_m input; V_bound input; out_iq_k_1 output; out_we_k_1 output; epsilon output; iq_out output; last_delta_uq input; iq_ref input; tau_ff input; res_uq output; res_ud output; judge_1 output; judge_2 output
function [out_delta_uq, out_delta_ud, iq_lb, iq_ub, out_iq_k_1, out_we_k_1, epsilon, iq_out, res_uq, res_ud, judge_1, judge_2] = fcn(we_k_1, we_k_2 , iq_k_1, iq_k_2, uq_k_1, ud_k_1,L_s, R_s, phi_m, V_bound, last_delta_uq,iq_ref, tau_ff)

delta_t = 0.001; %second
Inertial_Rotor = 0.03;
Npp = 21;
iq_max = 30;
delta_uq = 0;
delta_ud = 0;
stop_temp = 0;
delta_uq_gain = 1.0;
delta_iq_max = 5;
s = 1;
%% 对变化率进行clip
% if abs(iq_ref - iq_k_1) > delta_iq_max
%     iq_ref = iq_k_1 + sign(iq_ref)*delta_iq_max;
% end

% try integral, integral works.
filter = 0.2;
delta_uq = (uq_k_1 - (R_s * iq_k_1 + L_s * (iq_k_1 - iq_k_2)/delta_t + we_k_1* phi_m)) * filter + (1-filter) * last_delta_uq;
% delta_uq = uq_k_1 - (R_s * iq_k_1 + we_k_1* phi_m);
delta_ud = ud_k_1 - (-we_k_2 * L_s * iq_k_1);

res_uq = delta_uq;
res_ud = delta_ud;

% 只退阶u_d
% m = R_s + L_s / delta_t + (3* phi_m * phi_m * Npp* delta_t)/(2 *Inertial_Rotor);
% n = we_k_1 *phi_m - L_s /delta_t* iq_k_1 + delta_uq_gain * delta_uq - tau_ff * delta_t * phi_m / Inertial_Rotor;
% p = -we_k_1* L_s;

% u_q的速度也退阶
m = R_s + L_s / delta_t;
n = (we_k_1 + ((1.5*phi_m * iq_k_1 * Npp - tau_ff) / Inertial_Rotor) * 0.001 * s) *phi_m - L_s /delta_t* iq_k_1 + delta_uq_gain * delta_uq;
p = -we_k_1* L_s;


epsilon = 2*m*n*p*delta_ud + m*m*V_bound*V_bound + p*p*V_bound*V_bound - m*m*delta_ud*delta_ud - p*p*n*n;
epsilon_judgement_1 = sqrt(m*m+p*p)*V_bound - (m*delta_ud - p*n);
epsilon_judgement_2 = sqrt(m*m+p*p)*V_bound + m*delta_ud - p *n;
% ep_fake = (V_bound*sqrt(m*m+p*p))^2-(m*delta_ud - p*n)^2;
judge_1 = epsilon_judgement_1;
judge_2 = epsilon_judgement_2;

iq_lb_temp = 0;
iq_ub_temp = 0;
out_iq_k_1 = iq_k_1;
out_we_k_1 = we_k_1;
epsilon_less_than_0 = 0;

if epsilon >= 0
    iq_lb_temp = (-m*n - p*delta_ud - sqrt(epsilon)) / (m * m + p * p);
    iq_ub_temp = (-m*n - p* delta_ud +  sqrt(epsilon)) / (m * m + p * p);
    epsilon_less_than_0 = 0;
else
    epsilon_less_than_0 = 100;
end
%%

iq_lb = iq_lb_temp;
if(iq_lb > 0)
    iq_lb = 0;
end
iq_ub = iq_ub_temp;
if(iq_ub < 0)
    iq_ub = 0;
end

% Del's paper only consider the decelerate.
if (iq_ref * we_k_1) > 0 && (iq_ref > 0)
    % the same direction
    iq_lb = -35;
end

if (iq_ref * we_k_1) > 0 && (iq_ref < 0)
    % the same direction
    iq_ub = 35;
end

out_delta_uq = delta_uq;
out_delta_ud = delta_ud;
iq_out = max([iq_lb,min([iq_ref, iq_ub])]);

%% normal version
% m = R_s + L_s / delta_t + (3* phi_m * phi_m * Npp* delta_t)/(2 *Inertial_Rotor);
% n = we_k_1 *phi_m - L_s /delta_t* iq_k_1;
% p = -we_k_1* L_s;
% 
% epsilon = m* m* V_bound* V_bound - p* p* n* n + p* p* V_bound* V_bound;
% 
% iq_lb_temp = 0;
% iq_ub_temp = 0;
% out_iq_k_1 = iq_k_1;
% out_we_k_1 = we_k_1;
% 
% if epsilon >= 0
%     iq_lb_temp = (-m*n - sqrt(epsilon)) / (m * m + p * p);
%     iq_ub_temp = (-m*n + sqrt(epsilon)) / (m * m + p * p);
%     % if(iq_ub_temp > iq_max)
%     %     iq_ub_temp = iq_max;
%     % elseif (iq_lb_temp < -iq_max)
%     %     iq_lb_temp = -iq_max;
%     % end
% end

%% add res
% if stop == 0
%     delta_uq = uq_k_1 - (R_s * iq_k_1 + L_s * (iq_k_1 - iq_k_2)/delta_t + we_k_1* phi_m);
%     % delta_uq = uq_k_1 - (R_s * iq_k_1 + we_k_1* phi_m);
%     delta_ud = ud_k_1 - (-we_k_2 * L_s * iq_k_1);
% else
%     % delta_uq = last_delta_uq;
%     % delta_ud = last_delta_ud;
% end

== matlab function AJAC_Simulation/pre_alim ==
  settings: updateMethod=DISCRETE  sampleTime=0.001
  data: pvk_limit output; res_ud input; res_uq input; f data_store_memory; Ls input; phi_m input; Rs input; V_bound input; PVK_limit_last input; omega_k_1 input; iq_lb output; iq_ub output
function [pvk_limit, iq_lb, iq_ub]   = fcn(res_ud, res_uq, Ls, phi_m, Rs, V_bound, PVK_limit_last, omega_k_1)

delta_t = 0.001; %second
Inertial_Rotor = 0.03;
Npp = 21;
iq_max = 30;
steps = 1;

% try integral, integral works.

m = Rs;
n = omega_k_1 * phi_m + res_uq;
p = -omega_k_1* Ls;

epsilon = 2*m*n*p*res_ud + m*m*V_bound*V_bound + p*p*V_bound*V_bound - m*m*res_ud*res_ud - p*p*n*n;


iq_lb_temp = 0;
iq_ub_temp = 0;

if epsilon >= 0
    iq_lb_temp = (-m*n - p*res_ud - sqrt(epsilon)) / (m * m + p * p);
    iq_ub_temp = (-m*n - p* res_ud +  sqrt(epsilon)) / (m * m + p * p);
else
    
end
%%

iq_lb = iq_lb_temp;
if(iq_lb > 0)
    iq_lb = 0;
end
iq_ub = iq_ub_temp;
if(iq_ub < 0)
    iq_ub = 0;
end

% decelerate when omega < 0
pvk_limit_temp =0;
asym_filter = 0.1;
if (omega_k_1 >= 0)
    pvk_limit_temp = abs(iq_lb);
else
    pvk_limit_temp = abs(iq_ub);
end

if pvk_limit_temp < PVK_limit_last
    pvk_limit = pvk_limit_temp;
else
    pvk_limit = asym_filter * pvk_limit_temp + (1-asym_filter)*PVK_limit_last;
end

% if pvk_limit > iq_max
%     pvk_limit = iq_max
% end



% Del's paper only consider the decelerate.
% if (iq_ref * we_k_1) > 0 && (iq_ref > 0)
%     % the same direction
%     iq_lb = -25;
% end

% if (iq_ref * we_k_1) > 0 && (iq_ref < 0)
%     % the same direction
%     iq_ub = 25;
% end
% iq_out = max([iq_lb,min([iq_ref, iq_ub])]);

% epsilon_judgement_1 = sqrt(m*m+p*p)*V_bound - (m*delta_ud - p*n);
% epsilon_judgement_2 = sqrt(m*m+p*p)*V_bound + m*delta_ud - p *n;
% % ep_fake = (V_bound*sqrt(m*m+p*p))^2-(m*delta_ud - p*n)^2;
% judge_1 = epsilon_judgement_1;
% judge_2 = epsilon_judgement_2;

== matlab function AJAC_Simulation/Clark2 ==
  settings: updateMethod=DISCRETE  sampleTime=0.000025
  data: ia input; ialpha output; ib input; ic input; ibeta output
function [ialpha,ibeta] = fcn(ia,ib,ic)
ialpha = ia*2/3-(ib+ic)/3;
ibeta = (ib-ic)*sqrt(3)/3;

== matlab function AJAC_Simulation/Park2 ==
  settings: updateMethod=DISCRETE  sampleTime=0.000025
  data: iq output; ialpha input; ibeta input; theta input; id output
function [iq,id] = fcn(ialpha,ibeta,theta)
id = ialpha*cos(theta)+ibeta*sin(theta);
iq = -ialpha*sin(theta)+ibeta*cos(theta);

== matlab function AJAC_Simulation/QP ==
  settings: updateMethod=DISCRETE  sampleTime=0.001
  data: ddq output; epsilon output; tau_ref output; ddq_ref input; ddq_lb input; ddq_ub input; tau_lb input; tau_ub input; f data_store_memory; w1 input; w2 input; tau_ff input; last_tau_ref input
function [ddq, epsilon, tau_ref]  = fcn(ddq_ref, ddq_lb, ddq_ub, tau_lb, tau_ub, w1, w2, tau_ff, last_tau_ref)

inertial = 0.003;
tau_ref = 0;
ddq = 0;
epsilon = 0;
x0 = [0;0;last_tau_ref];
persistent opts;
if isempty(opts)
    opts = optimoptions('quadprog', ...
        'Display','off', ...
        'Algorithm','active-set'); % 常用且稳
end

H = [w1, 0,0;
    0, w2, 0;
    0, 0, 0;];
f = [-2*w1*ddq_ref;
    0;0];
A_eq = [-inertial, -1, 1];
B_eq = tau_ff;
%% comparision
lb_sf = [ddq_lb; -1000; tau_lb];
ub_sf = [ddq_ub; 1000; tau_ub];

%% normal
lb = [ddq_lb; -1000; -1000];
ub = [ddq_ub; 1000; 1000];

[x,~,exitflag] = quadprog(H,f,[],[],A_eq, B_eq, lb, ub, x0, opts);
if exitflag == 1
    ddq = x(1);
    epsilon = x(2);
    tau_ref = x(3);
end

== matlab function AJAC_Simulation/Capture_Dy_Motor_VK1 ==
  settings: updateMethod=DISCRETE  sampleTime=0.001
  data: res_uq output; res_ud output; we_k_1 input; we_k_2 input; iq_k_1 input; uq_k_1 input; ud_k_1 input; L_s input; R_s input; f data_store_memory; iq_lb output; iq_ub output; phi_m input; V_bound input; out_iq_k_1 output; out_we_k_1 output; epsilon output; iq_out output; last_delta_uq input; iq_ref input; tau_ff input
function [res_uq, res_ud,iq_lb, iq_ub, out_iq_k_1, out_we_k_1, epsilon, iq_out] = fcn(we_k_1, we_k_2 , iq_k_1, uq_k_1, ud_k_1,L_s, R_s, phi_m, V_bound, last_delta_uq,iq_ref, tau_ff)

delta_t = 0.001; %second
Inertial_Rotor = 0.0003;
Npp = 21;
iq_max = 30;
delta_uq = 0;
delta_ud = 0;
delta_uq_gain = 1.0;
steps = 100;

% try integral, integral works.
filter = 0.1;
delta_uq = (uq_k_1 - (R_s * iq_k_1 + we_k_1* phi_m)) * filter + (1-filter) * last_delta_uq;
% delta_uq = uq_k_1 - (R_s * iq_k_1 + we_k_1* phi_m);
delta_ud = ud_k_1 - (-we_k_2 * L_s * iq_k_1);

m = R_s + (3*phi_m*phi_m*Npp * steps * delta_t)/(2*Inertial_Rotor) + L_s / delta_t;
n = (we_k_1 - (tau_ff * delta_t * steps)/(Inertial_Rotor))*phi_m + delta_uq - L_s/delta_t * iq_k_1;
p = -we_k_1* L_s;

epsilon = 2*m*n*p*delta_ud + m*m*V_bound*V_bound + p*p*V_bound*V_bound - m*m*delta_ud*delta_ud - p*p*n*n;

iq_lb_temp = 0;
iq_ub_temp = 0;


if epsilon >= 0
    iq_lb_temp = (-m*n - p*delta_ud - sqrt(epsilon)) / (m * m + p * p);
    iq_ub_temp = (-m*n - p* delta_ud +  sqrt(epsilon)) / (m * m + p * p);
else
    
end
%%

iq_lb = iq_lb_temp;
if(iq_lb > 0)
    iq_lb = 0;
end
iq_ub = iq_ub_temp;
if(iq_ub < 0)
    iq_ub = 0;
end

out_iq_k_1 = iq_k_1;
out_we_k_1 = we_k_1;

% Del's paper only consider the decelerate.
% if (iq_ref * we_k_1) > 0 && (iq_ref > 0)
%     % the same direction
%     iq_lb = -25;
% end

% if (iq_ref * we_k_1) > 0 && (iq_ref < 0)
%     % the same direction
%     iq_ub = 25;
% end

res_uq = delta_uq;
res_ud = delta_ud;
iq_out = max([iq_lb,min([iq_ref, iq_ub])]);

== matlab function AJAC_Simulation/foc1 ==
  settings: updateMethod=DISCRETE  sampleTime=0.000025
  data: ud input; Tcmp1 output; uq input; theta input; Udc input; Tpwm input; Tcmp2 output; Tcmp3 output; sector output
function [Tcmp1,Tcmp2,Tcmp3,sector] = fcn(ud,uq,theta,Udc,Tpwm)
Valpha = ud*cos(theta) - uq*sin(theta);
Vbeta = ud*sin(theta) + uq*cos(theta);
AAR = Tpwm / 2;
%#codegen

sector = single(0);
Tcmp1 = single(0);
Tcmp2 = single(0);
Tcmp3 = single(0);

%========Parameters statement================

    Vref1 = Vbeta;							                   
    Vref2 = (sqrt(3)*Valpha - Vbeta)/2; 				    
    Vref3 = (-sqrt(3)*Valpha - Vbeta)/2;					
   
 %========Sector calculation=================

  if (Vref1>0)
	   sector = single(1);
  end
  if (Vref2>0)
	   sector = sector+single(2);
  end
  if (Vref3>0)
       sector = sector+single(4);
  end

%======== X Y Z calculation===================

X = sqrt(3)*Vbeta*Tpwm/(Udc*1.15);
Y = Tpwm/(Udc*1.15)*(3/2*Valpha+sqrt(3)/2*Vbeta);
Z = Tpwm/(Udc*1.15)*(-3/2*Valpha+sqrt(3)/2*Vbeta);	         

%==========Duty ratio calculation================
switch (sector)   
    case 1
        T1 = Z; T2 = Y; 
	case 2
        T1 = Y; T2 = -X; 
	case 3
        T1 = -Z; T2 = X; 
	case 4
        T1 = -X; T2 = Z;
	case 5
        T1 = X; T2 = -Y;
    otherwise
        T1 = -Y; T2 = -Z;
end

if T1+T2 > Tpwm
    T1 = T1/(T1+T2);
    T2 = T2/(T1+T2);
else
    T1 = T1;
    T2 = T2;
end

%ccr
ta = (Tpwm-(T1+T2))/4.0;
tb = ta+T1/2;
tc = tb+T2/2;

%%实际代码需要加上
%%ta = AAR -ta;
%%tb = AAR -tb;
%%tc = AAR -tc;

%==========Duty ratio calculation================
switch (sector)
    case 1 
        Tcmp1=tb;
        Tcmp2=ta;
        Tcmp3=tc; 
        
    case 2 
        Tcmp1=ta;
        Tcmp2=tc;
        Tcmp3=tb; 
       
    case 3 
        Tcmp1=ta;
        Tcmp2=tb;
        Tcmp3=tc; 
        
    case 4 
        Tcmp1=tc;
        Tcmp2=tb;
        Tcmp3=ta;
        
    case 5 
        Tcmp1=tc;
        Tcmp2=ta;
        Tcmp3=tb;
        
   case 6
       Tcmp1=tb;
       Tcmp2=tc;
       Tcmp3=ta;
end
end

== matlab function AJAC_Simulation/simplydecoupleud ==
  settings: updateMethod=DISCRETE  sampleTime=0.001
  data: res_uq output; res_ud output; we_k_1 input; we_k_2 input; iq_k_1 input; uq_k_1 input; ud_k_1 input; L_s input; R_s input; f data_store_memory; iq_lb output; iq_ub output; phi_m input; V_bound input; out_iq_k_1 output; out_we_k_1 output; epsilon output; iq_out output; last_delta_uq input; iq_ref input; tau_ff input
function [res_uq, res_ud,iq_lb, iq_ub, out_iq_k_1, out_we_k_1, epsilon, iq_out] = fcn(we_k_1, we_k_2 , iq_k_1, uq_k_1, ud_k_1,L_s, R_s, phi_m, V_bound, last_delta_uq,iq_ref, tau_ff)

delta_t = 0.001; %second
Inertial_Rotor = 0.0003;
Npp = 21;
iq_max = 30;
delta_uq = 0;
delta_ud = 0;
delta_uq_gain = 1.0;
steps = 100;

% try integral, integral works.
filter = 0.1;
delta_uq = (uq_k_1 - (R_s * iq_k_1 + we_k_1* phi_m)) * filter + (1-filter) * last_delta_uq;
% delta_uq = uq_k_1 - (R_s * iq_k_1 + we_k_1* phi_m);
delta_ud = ud_k_1 - (-we_k_2 * L_s * iq_k_1);

m = R_s + (3*phi_m*phi_m*Npp * steps * delta_t)/(2*Inertial_Rotor) + L_s / delta_t;
n = (we_k_1 - (tau_ff * delta_t * steps)/(Inertial_Rotor))*phi_m + delta_uq - L_s/delta_t * iq_k_1;
p = -we_k_1* L_s*iq_k_1+delta_ud;

epsilon = V_bound*V_bound - p*p;

iq_lb_temp = 0;
iq_ub_temp = 0;

if epsilon >= 0
    iq_lb_temp = (-n  - sqrt(epsilon)) / (m);
    iq_ub_temp = (-n  +  sqrt(epsilon)) / (m);
else
    
end
%%

iq_lb = iq_lb_temp;
if(iq_lb > 0)
    iq_lb = 0;
end
iq_ub = iq_ub_temp;
if(iq_ub < 0)
    iq_ub = 0;
end

out_iq_k_1 = iq_k_1;
out_we_k_1 = we_k_1;

% Del's paper only consider the decelerate.
% if (iq_ref * we_k_1) > 0 && (iq_ref > 0)
%     % the same direction
%     iq_lb = -25;
% end

% if (iq_ref * we_k_1) > 0 && (iq_ref < 0)
%     % the same direction
%     iq_ub = 25;
% end

res_uq = delta_uq;
res_ud = delta_ud;
iq_out = max([iq_lb,min([iq_ref, iq_ub])]);
